simulink model "lab_modulation_fm"  (R2023a)
settings: Solver=FixedStepDiscrete  StartTime=0.0  StopTime=1  FixedStep=0.0001  RelTol=1e-3
model workspace: external: MATLAB File lab_modulation_fm_saveas.m (data not in the file)
values from neighbouring files (symbols this model uses):
  variance = 0.01    [lab_modulation_fm_saveas.m]    (also in lab_modulation_pm_saveas.m = 0)
libraries: dspfdesign x2, dspmathops x1, commanapbnd3 x1
settings Model: Creator=andrey  LastModifiedBy=andrey
settings RTWCC: GPUComputeCapability=5.0

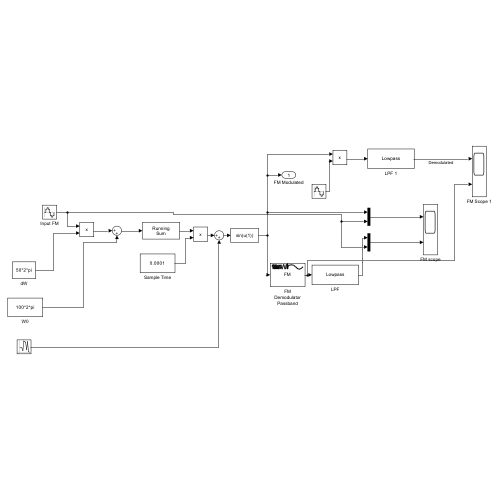
[thumbnail: Simulink's stored preview of the top-level diagram]
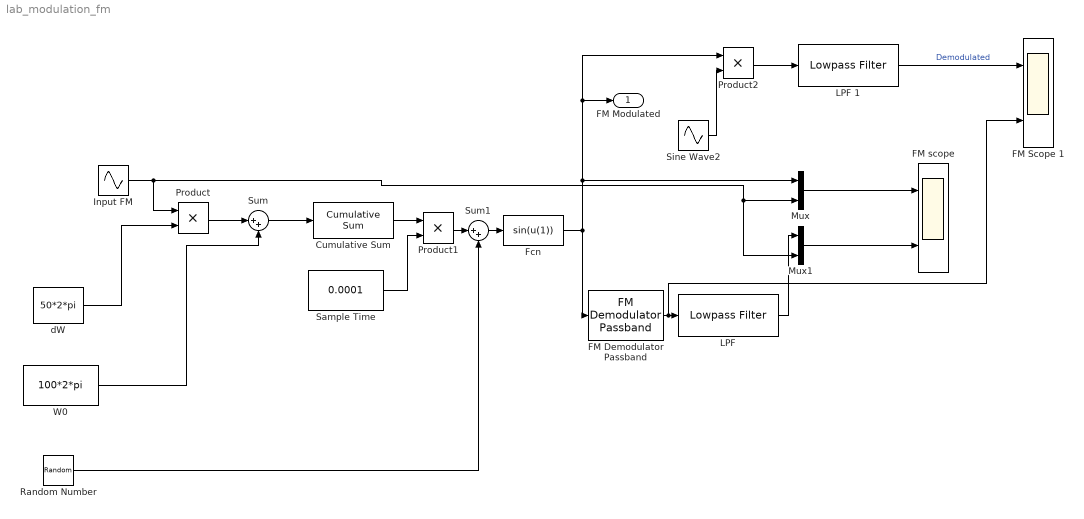
== system lab_modulation_fm ==
  Cumulative Sum : dspmathops/Cumulative Sum  dim=Channels (running sum)  InputProcessing=Columns as channels (frame based)  reset_popup=None  roundingMode=Floor  overflowMode=off  outputDataTypeStr=Inherit: Same as accumulator  outputMin=[]  outputMax=[]  outputLastDataTypeStr=Inherit: Same as accumulator
  FM Demodulator Passband : commanapbnd3/FM Demodulator Passband  Fc=100  Ph=0  Kc=frequencyDeviation  Ho=100
  FM Scope 1 : Scope  NumInputPorts=2
  FM scope : Scope  NumInputPorts=2
  Fcn : Fcn  Expr=sin(u(1))
  Input FM : Sin  Frequency=2*2*pi  SampleTime=0.0001
  LPF : dspfdesign/Lowpass Filter  FilterType=FIR  DesignForMinimumOrder=on  FilterOrder=50  PassbandFrequency=0.1  StopbandFrequency=100  PassbandRipple=0.1  StopbandAttenuation=80  SampleRate=44100  SimulateUsing=Interpreted execution  roundingMode=Floor  coeffsDataTypeStr=fixdt(1,16)
  LPF 1 : dspfdesign/Lowpass Filter  FilterType=FIR  DesignForMinimumOrder=on  FilterOrder=50  PassbandFrequency=10  StopbandFrequency=100  PassbandRipple=0.1  StopbandAttenuation=80  SampleRate=44100  SimulateUsing=Interpreted execution  roundingMode=Floor  coeffsDataTypeStr=fixdt(1,16)
  Mux : Mux  Inputs=2
  Mux1 : Mux  Inputs=2
  Product : Product
  Product1 : Product
  Product2 : Product
  Random Number : RandomNumber  Variance=variance  SampleTime=0.1
  Sample Time : Constant  Value=0.0001
  Sine Wave2 : Sin  Frequency=100*2*pi  SampleTime=0.0001
  Sum : Sum  Inputs=|++
  Sum1 : Sum  Inputs=|++
  W0 : Constant  Value=100*2*pi
  dW : Constant  Value=50*2*pi
  FM Modulated : Outport
  wires:
  Sine Wave2/1 -> Product2/2
  Product2/1 -> LPF 1/1
  LPF 1/1 -> FM Scope 1/1  "Demodulated"
  Mux1/1 -> FM scope/2
  Mux/1 -> FM scope/1
  Input FM/1 -> Mux/2, Mux1/2, Product/1
  FM Demodulator Passband/1 -> FM Scope 1/2, LPF/1
  LPF/1 -> Mux1/1
  dW/1 -> Product/2
  W0/1 -> Sum/2
  Product/1 -> Sum/1
  Sum/1 -> Cumulative Sum/1
  Sample Time/1 -> Product1/2
  Fcn/1 -> FM Demodulator Passband/1, Product2/1, FM Modulated/1, Mux/1
  Cumulative Sum/1 -> Product1/1
  Product1/1 -> Sum1/1
  Sum1/1 -> Fcn/1
  Random Number/1 -> Sum1/2
